simulink model "EMI_SC01B_R2_Halfbridge"  (R2026a)
settings: Solver=FixedStepDiscrete  StopTime=5.0000000000000004e-06  FixedStep=5.0000000000000003e-10  RelTol=1.0000000000000001e-05  AbsTol=1.0000000000000001e-09
model workspace (MAT data in the model file):
  sc01bGateHigh = timeseries
  sc01bGateHigh.Name = 'unnamed'
  sc01bGateHigh.DataInfo = tsdata.datametadata
  sc01bGateHigh.DataInfo.Interpolation = tsdata.interpolation
  sc01bGateHigh.DataInfo.Interpolation.Fhandle : function handle (value not decoded)
  sc01bGateHigh.DataInfo.Interpolation.Name = 'linear'
  sc01bGateHigh.TimeInfo = tsdata.timemetadata
  sc01bGateHigh.TimeInfo.Length = 10
  sc01bGateHigh.TimeInfo.DuplicateTimes = 0
  sc01bGateHigh.TimeInfo.Time_ = [0; 2.019e-06; 2.039e-06; 2.32e-06; 2.34e-06; 3.719e-06; 3.739e-06; 4.02e-06; 4.04e-06; 5e-06]
  sc01bGateHigh.TimeInfo.Initialized = 1
  sc01bGateHigh.QualityInfo = tsdata.qualmetadata
  sc01bGateHigh.Data_ = [12; 12; -1.5; -1.5; -1.5; -1.5; -1.5; -1.5; 12; 12]
  sc01bGateLow = timeseries
  sc01bGateLow.Name = 'unnamed'
  sc01bGateLow.DataInfo = tsdata.datametadata
  sc01bGateLow.DataInfo.Interpolation = tsdata.interpolation
  sc01bGateLow.DataInfo.Interpolation.Fhandle : function handle (value not decoded)
  sc01bGateLow.DataInfo.Interpolation.Name = 'linear'
  sc01bGateLow.TimeInfo = tsdata.timemetadata
  sc01bGateLow.TimeInfo.Length = 10
  sc01bGateLow.TimeInfo.DuplicateTimes = 0
  sc01bGateLow.TimeInfo.Time_ = [0; 2.019e-06; 2.039e-06; 2.32e-06; 2.34e-06; 3.719e-06; 3.739e-06; 4.02e-06; 4.04e-06; 5e-06]
  sc01bGateLow.TimeInfo.Initialized = 1
  sc01bGateLow.QualityInfo = tsdata.qualmetadata
  sc01bGateLow.Data_ = [-1.5; -1.5; -1.5; -1.5; 12; 12; -1.5; -1.5; -1.5; -1.5]
  sc01bParams.meta.id = "SC01B-R2-IAUC100N04S6L014"
  sc01bParams.meta.case = "nominal"
  sc01bParams.meta.scope = "Isothermal device-model verification; no physical source validation"
  sc01bParams.device.series = "Infineon OptiMOS6 40V"
  sc01bParams.device.name = "IAUC100N04S6L014"
  sc01bParams.device.temperature_C = 25
  sc01bParams.device.voltageRating_V = 40
  sc01bParams.device.gateRating_V = 16
  sc01bParams.device.source = "MATLAB R2026a shipped Infineon SPICE model, typical parameters"
  sc01bParams.bus.voltage_V = 24
  sc01bParams.bus.feedResistance_Ohm = 0.05
  sc01bParams.bus.feedInductance_H = 2e-08
  sc01bParams.bus.capacitance_F = 1e-05
  sc01bParams.bus.capacitorESR_Ohm = 0.01
  sc01bParams.bus.provenance = "Assumed bench supply and local decoupling, not selected layout or capacitor"
  sc01bParams.load.inductance_H = 0.0025
  sc01bParams.load.resistance_Ohm = 8
  sc01bParams.load.referenceCurrent_A = 3
  sc01bParams.load.provenance = "Assumed8ohm/2.5mH load; high-side initiallyON, consistentDC operating point near3A; current follows circuit equations"
  sc01bParams.driver.reference = "Revised bipolar behavioral driver with directional gate impedance; not UCC27211A-equivalent"
  sc01bParams.driver.voltage_V = 12
  sc01bParams.driver.outputResistance_Ohm = 3
  sc01bParams.driver.externalResistance_Ohm = 22
  sc01bParams.driver.additionalTurnOnResistance_Ohm = 0
  sc01bParams.driver.turnOffResistance_Ohm = 3
  sc01bParams.driver.offVoltage_V = -1.5
  sc01bParams.driver.riseDelay_s = 2e-08
  sc01bParams.driver.fallDelay_s = 1.9e-08
  sc01bParams.driver.commandRamp_s = 2e-08
  sc01bParams.driver.provenance = "R2 assumes 12V on/-1.5V off regulated floating supplies and unequal charge/discharge impedance. Ron=3ohm+external gate resistor; total Roff=3ohm. The original 20/19ns delays,20ns linear ramps,and300ns deadtime are retained. Negative rail and split-output behavior are explicit design changes; no complete driver IC, current limit, clamp diode dynamics, or bootstrap dynamics are modeled."
  sc01bParams.control.highOn_s = 4e-06
  sc01bParams.control.highOff_s = 2e-06
  sc01bParams.control.initialHigh = 1
  sc01bParams.control.deadTime_s = 3e-07
  sc01bParams.control.provenance = "Assumed high-side off/on commutation pair with complementary low-side operation; dead time commanded before driver delay"
  sc01bParams.simulation.stopTime_s = 5e-06
  sc01bParams.simulation.maxStep_s = 5e-10
  sc01bParams.simulation.relativeTolerance = 1e-05
  sc01bParams.simulation.absoluteTolerance = 1e-09
  sc01bParams.validation.startTime_s = 1e-06
  sc01bParams.validation.provenance = "Exclude initialization preamble from edge comparison; separately report initial and pre-edge current"
  sc01bSchema = 4
undefined symbols (not defined in the file): ee
libraries: fl_lib x24, nesl_utility x17, sc01b_driver_lib x2
settings Model: Creator=adand  LastModifiedBy=adand
settings DebuggingCC: MinStepSizeMsg=error
settings SimscapeCC: SimscapeLogName=sc01bSimlog  SimscapeLogLimitData=off

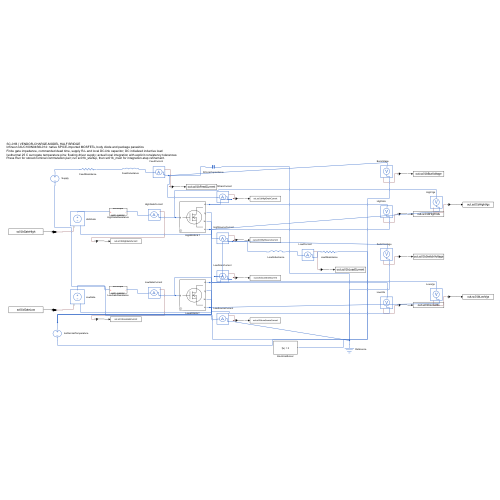
[thumbnail: Simulink's stored preview of the top-level diagram]
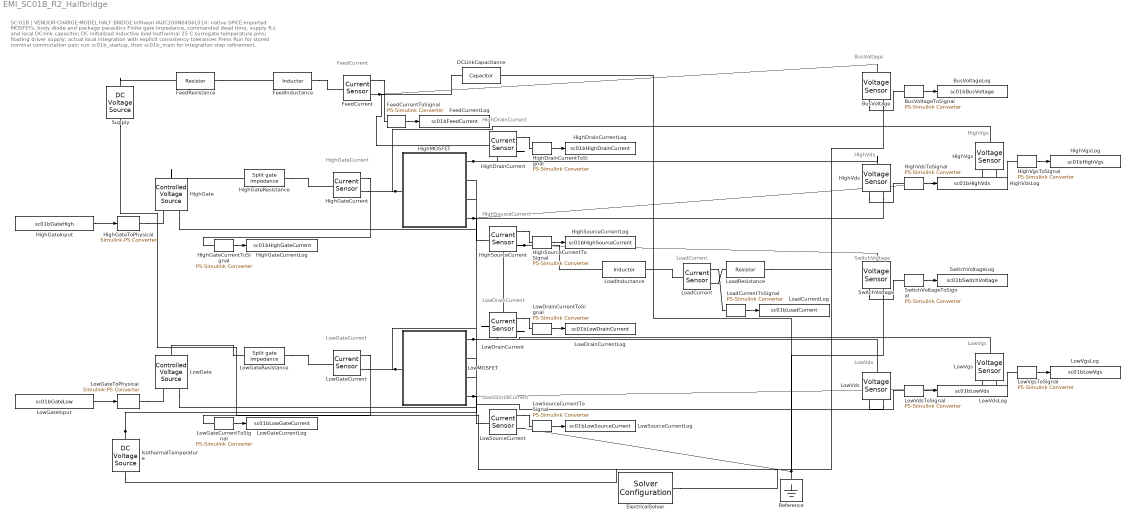
== system EMI_SC01B_R2_Halfbridge ==
  note: FeedCurrent
  note: HighDrainCurrent
  note: HighSourceCurrent
  note: LowDrainCurrent
  note: LowSourceCurrent
  note: HighGateCurrent
  note: LowGateCurrent
  note: LoadCurrent
  note: SwitchVoltage
  note: BusVoltage
  note: HighVgs
  note: HighVds
  note: LowVgs
  note: LowVds
  note: SC-01B | VENDOR-CHARGE-MODEL HALF BRIDGE
      | Infineon IAUC100N04S6L014: native SPICE-imported MOSFETs, body diode and package parasitics
      | Finite gate impedance, commanded dead time, supply R-L and local DC-link capacitor; DC initialized inductive load
      | Isothermal 25 C surrogate temperature pins; floating driver supply; actual local integration with explicit consistency tolerances
      | Press Run for stored nominal commutation pair; run sc01b_startup, then sc01b_main for integration-step refinement.
  BusVoltage : fl_lib/Electrical/Electrical Sensors/Voltage Sensor
  BusVoltageLog : ToWorkspace  VariableName=sc01bBusVoltage  SaveFormat=Timeseries  SampleTime=-1
  BusVoltageToSignal : nesl_utility/PS-Simulink Converter  PhysicalDomain=network_engine_domain  SubClassName=ps_output  LeftPortType=input  RightPortType=output  PseudoPeriodic=off  Frequencies=[]  VectorFormat=inherit  Unit=V  AffineConversion=off
  DCLinkCapacitance : fl_lib/Electrical/Electrical Elements/Capacitor  c=sc01bParams.bus.capacitance_F F  r=sc01bParams.bus.capacitorESR_Ohm Ohm  g=0 1/Ohm  i_specify=off  i_priority=None  i=0 A  i_nominal_specify=off  i_nominal_value=1  i_nominal_unit=A  v_specify=off  v_priority=None  v=0 V  v_nominal_specify=off  v_nominal_value=1  v_nominal_unit=V  vc_specify=off  vc_priority=High  vc=0 V  vc_nominal_specify=off  vc_nominal_value=1  vc_nominal_unit=V
  ElectricalSolver : nesl_utility/Solver Configuration  PhysicalDomain=network_engine_domain  SubClassName=solver  LeftPortType=input  RightPortType=generic  Tones=[]  Harmonics=[]  SimulateNoise=off  Profile=off  UseLocalSampling=off  EnableSwitchedLinearOptims=on  FrequencyDomain=off  UseCCode=off  RelTol=0.001  AbsTol=0.001  MinStep=1e-09  ToWorkspace=off  RevertToSquareIcSolve=off  NumHomotopyIterations=100  PhasorMode=off  PhasorModeNumHarmonics=1  ConsistencySolver=NEWTON_XTOL_AFTER_FTOL  CanonicalOrdering=CANONICAL  OptimizeIntermediates=OPTIMIZED  IndexReductionMethod=DerivativeReplacement  DoDC=on  ResidualTolerance=1e-09  ConsistencyTolSource=LOCAL  ConsistencyAbsTol=9.9999999999999998e-13  ConsistencyRelTol=1e-08  ConsistencyTolFactor=1  UseLocalSolver=on  LocalSolverChoice=NE_TRAPEZOIDAL_ADVANCER  ResolveIndetEquations=on  FunctionEvalNumThread=1  LocalSolverSampleTime=5.0000000000000003e-10  DoFixedCost=off  MaxNonlinIter=3  MaxModeIter=2  ComputeImpulses=off  ImpulseIterations=2  LinearAlgebra=auto  LinearAlgebraNumThread=0  EquationFormulation=NE_TIME_EF  DelaysMemoryBudget=1024  AutomaticFiltering=off  FilteringTimeConstant=0.001  PartitionStorageMethod=AS_NEEDED  PartitionMemoryBudget=1024  PartitionMethod=ROBUST  MultibodyUseLocalSolver=off  MultibodyLocalSolverChoice=ODE1  MultibodyLocalSolverSampleTime=0.001
  FeedCurrent : fl_lib/Electrical/Electrical Sensors/Current Sensor
  FeedCurrentLog : ToWorkspace  VariableName=sc01bFeedCurrent  SaveFormat=Timeseries  SampleTime=-1
  FeedCurrentToSignal : nesl_utility/PS-Simulink Converter  PhysicalDomain=network_engine_domain  SubClassName=ps_output  LeftPortType=input  RightPortType=output  PseudoPeriodic=off  Frequencies=[]  VectorFormat=inherit  Unit=A  AffineConversion=off
  FeedInductance : fl_lib/Electrical/Electrical Elements/Inductor  l=sc01bParams.bus.feedInductance_H H  r=0 Ohm  g=0 1/Ohm  i_specify=off  i_priority=None  i=0 A  i_nominal_specify=off  i_nominal_value=1  i_nominal_unit=A  v_specify=off  v_priority=None  v=0 V  v_nominal_specify=off  v_nominal_value=1  v_nominal_unit=V  i_L_specify=off  i_L_priority=High  i_L=0 A  i_L_nominal_specify=off  i_L_nominal_value=1  i_L_nominal_unit=A
  FeedResistance : fl_lib/Electrical/Electrical Elements/Resistor  R=sc01bParams.bus.feedResistance_Ohm Ohm  i_specify=off  i_priority=None  i=0 A  i_nominal_specify=off  i_nominal_value=1  i_nominal_unit=A  v_specify=off  v_priority=None  v=0 V  v_nominal_specify=off  v_nominal_value=1  v_nominal_unit=V
  HighDrainCurrent : fl_lib/Electrical/Electrical Sensors/Current Sensor
  HighDrainCurrentLog : ToWorkspace  VariableName=sc01bHighDrainCurrent  SaveFormat=Timeseries  SampleTime=-1
  HighDrainCurrentToSignal : nesl_utility/PS-Simulink Converter  PhysicalDomain=network_engine_domain  SubClassName=ps_output  LeftPortType=input  RightPortType=output  PseudoPeriodic=off  Frequencies=[]  VectorFormat=inherit  Unit=A  AffineConversion=off
  HighGate : fl_lib/Electrical/Electrical Sources/Controlled Voltage Source
  HighGateCurrent : fl_lib/Electrical/Electrical Sensors/Current Sensor
  HighGateCurrentLog : ToWorkspace  VariableName=sc01bHighGateCurrent  SaveFormat=Timeseries  SampleTime=-1
  HighGateCurrentToSignal : nesl_utility/PS-Simulink Converter  PhysicalDomain=network_engine_domain  SubClassName=ps_output  LeftPortType=input  RightPortType=output  PseudoPeriodic=off  Frequencies=[]  VectorFormat=inherit  Unit=A  AffineConversion=off
  HighGateInput : FromWorkspace  VariableName=sc01bGateHigh  OutputAfterFinalValue=Holding final value
  HighGateResistance : sc01b_driver_lib/Split gate impedance  Ron=sc01bParams.driver.outputResistance_Ohm+sc01bParams.driver.externalResistance_Ohm+sc01bParams.driver.additionalTurnOnResistance_Ohm Ohm  Roff=sc01bParams.driver.turnOffResistance_Ohm Ohm  i_specify=off  i_priority=None  i=0 A  i_nominal_specify=off  i_nominal_value=1  i_nominal_unit=A  v_specify=off  v_priority=None  v=0 V  v_nominal_specify=off  v_nominal_value=1  v_nominal_unit=V
  HighGateToPhysical : nesl_utility/Simulink-PS Converter  PhysicalDomain=network_engine_domain  SubClassName=ps_input  LeftPortType=input  RightPortType=output  PseudoPeriodic=off  Frequencies=[]  NoiseDistribution=none  NoiseParameters=[]  Unit=V  AffineConversion=off  FilteringAndDerivatives=provide  SimscapeFilterOrder=1  InputFilterTimeConstant=0.001  UdotUserProvided=0
  HighMOSFET : Subsystem  LoadFcn=ee.forwardingCallback();  mask(SPICE-Imported MOSFET){SeriesChoice=Infineon OptiMOS6 40V, DeviceChoice=IAUC100N04S6L014}
      mask prompts: SeriesChoice "physmod:ee:spiceimportedmosfet:Series_MP"; DeviceChoice "physmod:ee:spiceimportedmosfet:Device_MP"
      mask help: physmod:ee:spiceimportedmosfet:SPICEimportedMOSFETblock_MD
      mask init:
      | ee.internal.spice.maskInitialization(gcb)
      settings: CopyFcn=set_param(gcb,'LinkStatus','none');
      mask Help: helpview('sps','spice-imported-mosfet-block')
      mask TypeOptions SeriesChoice: Infineon OptiMOS7 40V | Infineon OptiMOS6 40V | Infineon OptiMOS5 60V | Infineon OptiMOS4 60V | Infineon OptiMOS7 80V | Infineon OptiMOS5 80V | Infineon OptiMOS7 100V | Infineon OptiMOS5 100V | Infineon OptiMOS5 120V | Infineon OptiMOST 120V
      mask Callback SeriesChoice:
      | %Run mask initialization to update the block help
      | ee.internal.spice.seriesCallback(gcb)
      mask TypeOptions DeviceChoice: IAUC60N04S6L039 | IAUC60N04S6N044 | IAUC80N04S6L032 | IAUC80N04S6N036 | IAUC100N04S6L014 | IAUC100N04S6L020 | IAUC100N04S6L025 | IAUC100N04S6N015 | IAUC100N04S6N022 | IAUC100N04S6N028 | IAUC120N04S6L008 | IAUC120N04S6L009 | IAUC120N04S6L012 | IAUC120N04S6N009 | IAUC120N04S6N010 | IAUC120N04S6N013
      mask DialogControl ParameterGroupVar Prompt: physmod:ee:spiceimportedmosfet:DeviceSelection_MH
      mask DialogControl SeriesChoice Prompt: Series
      mask DialogControl DeviceChoice Prompt: Device
  HighSourceCurrent : fl_lib/Electrical/Electrical Sensors/Current Sensor
  HighSourceCurrentLog : ToWorkspace  VariableName=sc01bHighSourceCurrent  SaveFormat=Timeseries  SampleTime=-1
  HighSourceCurrentToSignal : nesl_utility/PS-Simulink Converter  PhysicalDomain=network_engine_domain  SubClassName=ps_output  LeftPortType=input  RightPortType=output  PseudoPeriodic=off  Frequencies=[]  VectorFormat=inherit  Unit=A  AffineConversion=off
  HighVds : fl_lib/Electrical/Electrical Sensors/Voltage Sensor
  HighVdsLog : ToWorkspace  VariableName=sc01bHighVds  SaveFormat=Timeseries  SampleTime=-1
  HighVdsToSignal : nesl_utility/PS-Simulink Converter  PhysicalDomain=network_engine_domain  SubClassName=ps_output  LeftPortType=input  RightPortType=output  PseudoPeriodic=off  Frequencies=[]  VectorFormat=inherit  Unit=V  AffineConversion=off
  HighVgs : fl_lib/Electrical/Electrical Sensors/Voltage Sensor
  HighVgsLog : ToWorkspace  VariableName=sc01bHighVgs  SaveFormat=Timeseries  SampleTime=-1
  HighVgsToSignal : nesl_utility/PS-Simulink Converter  PhysicalDomain=network_engine_domain  SubClassName=ps_output  LeftPortType=input  RightPortType=output  PseudoPeriodic=off  Frequencies=[]  VectorFormat=inherit  Unit=V  AffineConversion=off
  IsothermalTemperature : fl_lib/Electrical/Electrical Sources/DC Voltage Source  v0=sc01bParams.device.temperature_C V
  LoadCurrent : fl_lib/Electrical/Electrical Sensors/Current Sensor
  LoadCurrentLog : ToWorkspace  VariableName=sc01bLoadCurrent  SaveFormat=Timeseries  SampleTime=-1
  LoadCurrentToSignal : nesl_utility/PS-Simulink Converter  PhysicalDomain=network_engine_domain  SubClassName=ps_output  LeftPortType=input  RightPortType=output  PseudoPeriodic=off  Frequencies=[]  VectorFormat=inherit  Unit=A  AffineConversion=off
  LoadInductance : fl_lib/Electrical/Electrical Elements/Inductor  l=sc01bParams.load.inductance_H H  r=0 Ohm  g=0 1/Ohm  i_specify=off  i_priority=None  i=0 A  i_nominal_specify=off  i_nominal_value=1  i_nominal_unit=A  v_specify=off  v_priority=None  v=0 V  v_nominal_specify=off  v_nominal_value=1  v_nominal_unit=V  i_L_specify=off  i_L_priority=High  i_L=0 A  i_L_nominal_specify=off  i_L_nominal_value=1  i_L_nominal_unit=A
  LoadResistance : fl_lib/Electrical/Electrical Elements/Resistor  R=sc01bParams.load.resistance_Ohm Ohm  i_specify=off  i_priority=None  i=0 A  i_nominal_specify=off  i_nominal_value=1  i_nominal_unit=A  v_specify=off  v_priority=None  v=0 V  v_nominal_specify=off  v_nominal_value=1  v_nominal_unit=V
  LowDrainCurrent : fl_lib/Electrical/Electrical Sensors/Current Sensor
  LowDrainCurrentLog : ToWorkspace  VariableName=sc01bLowDrainCurrent  SaveFormat=Timeseries  SampleTime=-1
  LowDrainCurrentToSignal : nesl_utility/PS-Simulink Converter  PhysicalDomain=network_engine_domain  SubClassName=ps_output  LeftPortType=input  RightPortType=output  PseudoPeriodic=off  Frequencies=[]  VectorFormat=inherit  Unit=A  AffineConversion=off
  LowGate : fl_lib/Electrical/Electrical Sources/Controlled Voltage Source
  LowGateCurrent : fl_lib/Electrical/Electrical Sensors/Current Sensor
  LowGateCurrentLog : ToWorkspace  VariableName=sc01bLowGateCurrent  SaveFormat=Timeseries  SampleTime=-1
  LowGateCurrentToSignal : nesl_utility/PS-Simulink Converter  PhysicalDomain=network_engine_domain  SubClassName=ps_output  LeftPortType=input  RightPortType=output  PseudoPeriodic=off  Frequencies=[]  VectorFormat=inherit  Unit=A  AffineConversion=off
  LowGateInput : FromWorkspace  VariableName=sc01bGateLow  OutputAfterFinalValue=Holding final value
  LowGateResistance : sc01b_driver_lib/Split gate impedance  Ron=sc01bParams.driver.outputResistance_Ohm+sc01bParams.driver.externalResistance_Ohm+sc01bParams.driver.additionalTurnOnResistance_Ohm Ohm  Roff=sc01bParams.driver.turnOffResistance_Ohm Ohm  i_specify=off  i_priority=None  i=0 A  i_nominal_specify=off  i_nominal_value=1  i_nominal_unit=A  v_specify=off  v_priority=None  v=0 V  v_nominal_specify=off  v_nominal_value=1  v_nominal_unit=V
  LowGateToPhysical : nesl_utility/Simulink-PS Converter  PhysicalDomain=network_engine_domain  SubClassName=ps_input  LeftPortType=input  RightPortType=output  PseudoPeriodic=off  Frequencies=[]  NoiseDistribution=none  NoiseParameters=[]  Unit=V  AffineConversion=off  FilteringAndDerivatives=provide  SimscapeFilterOrder=1  InputFilterTimeConstant=0.001  UdotUserProvided=0
  LowMOSFET : Subsystem  LoadFcn=ee.forwardingCallback();  mask(SPICE-Imported MOSFET){SeriesChoice=Infineon OptiMOS6 40V, DeviceChoice=IAUC100N04S6L014}
      mask prompts: SeriesChoice "physmod:ee:spiceimportedmosfet:Series_MP"; DeviceChoice "physmod:ee:spiceimportedmosfet:Device_MP"
      mask help: physmod:ee:spiceimportedmosfet:SPICEimportedMOSFETblock_MD
      mask init:
      | ee.internal.spice.maskInitialization(gcb)
      settings: CopyFcn=set_param(gcb,'LinkStatus','none');
      mask Help: helpview('sps','spice-imported-mosfet-block')
      mask TypeOptions SeriesChoice: Infineon OptiMOS7 40V | Infineon OptiMOS6 40V | Infineon OptiMOS5 60V | Infineon OptiMOS4 60V | Infineon OptiMOS7 80V | Infineon OptiMOS5 80V | Infineon OptiMOS7 100V | Infineon OptiMOS5 100V | Infineon OptiMOS5 120V | Infineon OptiMOST 120V
      mask Callback SeriesChoice:
      | %Run mask initialization to update the block help
      | ee.internal.spice.seriesCallback(gcb)
      mask TypeOptions DeviceChoice: IAUC60N04S6L039 | IAUC60N04S6N044 | IAUC80N04S6L032 | IAUC80N04S6N036 | IAUC100N04S6L014 | IAUC100N04S6L020 | IAUC100N04S6L025 | IAUC100N04S6N015 | IAUC100N04S6N022 | IAUC100N04S6N028 | IAUC120N04S6L008 | IAUC120N04S6L009 | IAUC120N04S6L012 | IAUC120N04S6N009 | IAUC120N04S6N010 | IAUC120N04S6N013
      mask DialogControl ParameterGroupVar Prompt: physmod:ee:spiceimportedmosfet:DeviceSelection_MH
      mask DialogControl SeriesChoice Prompt: Series
      mask DialogControl DeviceChoice Prompt: Device
  LowSourceCurrent : fl_lib/Electrical/Electrical Sensors/Current Sensor
  LowSourceCurrentLog : ToWorkspace  VariableName=sc01bLowSourceCurrent  SaveFormat=Timeseries  SampleTime=-1
  LowSourceCurrentToSignal : nesl_utility/PS-Simulink Converter  PhysicalDomain=network_engine_domain  SubClassName=ps_output  LeftPortType=input  RightPortType=output  PseudoPeriodic=off  Frequencies=[]  VectorFormat=inherit  Unit=A  AffineConversion=off
  LowVds : fl_lib/Electrical/Electrical Sensors/Voltage Sensor
  LowVdsLog : ToWorkspace  VariableName=sc01bLowVds  SaveFormat=Timeseries  SampleTime=-1
  LowVdsToSignal : nesl_utility/PS-Simulink Converter  PhysicalDomain=network_engine_domain  SubClassName=ps_output  LeftPortType=input  RightPortType=output  PseudoPeriodic=off  Frequencies=[]  VectorFormat=inherit  Unit=V  AffineConversion=off
  LowVgs : fl_lib/Electrical/Electrical Sensors/Voltage Sensor
  LowVgsLog : ToWorkspace  VariableName=sc01bLowVgs  SaveFormat=Timeseries  SampleTime=-1
  LowVgsToSignal : nesl_utility/PS-Simulink Converter  PhysicalDomain=network_engine_domain  SubClassName=ps_output  LeftPortType=input  RightPortType=output  PseudoPeriodic=off  Frequencies=[]  VectorFormat=inherit  Unit=V  AffineConversion=off
  Reference : fl_lib/Electrical/Electrical Elements/Electrical Reference
  Supply : fl_lib/Electrical/Electrical Sources/DC Voltage Source  v0=sc01bParams.bus.voltage_V V
  SwitchVoltage : fl_lib/Electrical/Electrical Sensors/Voltage Sensor
  SwitchVoltageLog : ToWorkspace  VariableName=sc01bSwitchVoltage  SaveFormat=Timeseries  SampleTime=-1
  SwitchVoltageToSignal : nesl_utility/PS-Simulink Converter  PhysicalDomain=network_engine_domain  SubClassName=ps_output  LeftPortType=input  RightPortType=output  PseudoPeriodic=off  Frequencies=[]  VectorFormat=inherit  Unit=V  AffineConversion=off
  wires:
  HighGateInput/1 -> HighGateToPhysical/1
  LowGateInput/1 -> LowGateToPhysical/1
  FeedCurrentToSignal/1 -> FeedCurrentLog/1
  HighDrainCurrentToSignal/1 -> HighDrainCurrentLog/1
  HighSourceCurrentToSignal/1 -> HighSourceCurrentLog/1
  LowDrainCurrentToSignal/1 -> LowDrainCurrentLog/1
  LowSourceCurrentToSignal/1 -> LowSourceCurrentLog/1
  HighGateCurrentToSignal/1 -> HighGateCurrentLog/1
  LowGateCurrentToSignal/1 -> LowGateCurrentLog/1
  LoadCurrentToSignal/1 -> LoadCurrentLog/1
  SwitchVoltageToSignal/1 -> SwitchVoltageLog/1
  BusVoltageToSignal/1 -> BusVoltageLog/1
  HighVgsToSignal/1 -> HighVgsLog/1
  HighVdsToSignal/1 -> HighVdsLog/1
  LowVgsToSignal/1 -> LowVgsLog/1
  LowVdsToSignal/1 -> LowVdsLog/1
  connections:
  HighGateToPhysical/RConn1 -- HighGate/RConn1
  LowGateToPhysical/RConn1 -- LowGate/RConn1
  FeedCurrent/RConn1 -- FeedCurrentToSignal/LConn1
  HighDrainCurrent/RConn1 -- HighDrainCurrentToSignal/LConn1
  HighSourceCurrent/RConn1 -- HighSourceCurrentToSignal/LConn1
  LowDrainCurrent/RConn1 -- LowDrainCurrentToSignal/LConn1
  LowSourceCurrent/RConn1 -- LowSourceCurrentToSignal/LConn1
  HighGateCurrent/RConn1 -- HighGateCurrentToSignal/LConn1
  LowGateCurrent/RConn1 -- LowGateCurrentToSignal/LConn1
  LoadCurrent/RConn1 -- LoadCurrentToSignal/LConn1
  SwitchVoltage/RConn1 -- SwitchVoltageToSignal/LConn1
  BusVoltage/RConn1 -- BusVoltageToSignal/LConn1
  HighVgs/RConn1 -- HighVgsToSignal/LConn1
  HighVds/RConn1 -- HighVdsToSignal/LConn1
  LowVgs/RConn1 -- LowVgsToSignal/LConn1
  LowVds/RConn1 -- LowVdsToSignal/LConn1
  Supply/LConn1 -- FeedResistance/LConn1
  FeedResistance/RConn1 -- FeedInductance/LConn1
  FeedInductance/RConn1 -- FeedCurrent/LConn1
  DCLinkCapacitance/LConn1 -- FeedCurrent/RConn2 -- HighDrainCurrent/LConn1 -- BusVoltage/LConn1
  DCLinkCapacitance/RConn1 -- Reference/LConn1 -- LowSourceCurrent/RConn2 -- LoadResistance/RConn1 -- Supply/RConn1 -- IsothermalTemperature/RConn1 -- ElectricalSolver/RConn1 -- SwitchVoltage/RConn2 -- BusVoltage/RConn2
  HighMOSFET/RConn1 -- HighDrainCurrent/RConn2 -- HighVds/LConn1
  HighSourceCurrent/LConn1 -- HighMOSFET/RConn4 -- HighGate/RConn2 -- HighVgs/RConn2 -- HighVds/RConn2
  LowDrainCurrent/LConn1 -- HighSourceCurrent/RConn2 -- LoadInductance/LConn1 -- SwitchVoltage/LConn1
  LowMOSFET/RConn1 -- LowDrainCurrent/RConn2 -- LowVds/LConn1
  LowSourceCurrent/LConn1 -- LowMOSFET/RConn4 -- LowGate/RConn2 -- LowVgs/RConn2 -- LowVds/RConn2
  LoadInductance/RConn1 -- LoadCurrent/LConn1
  LoadCurrent/RConn2 -- LoadResistance/LConn1
  HighGate/LConn1 -- HighGateResistance/LConn1
  HighGateResistance/RConn1 -- HighGateCurrent/LConn1
  HighMOSFET/LConn1 -- HighGateCurrent/RConn2 -- HighVgs/LConn1
  HighMOSFET/RConn2 -- IsothermalTemperature/LConn1 -- HighMOSFET/RConn3 -- LowMOSFET/RConn2 -- LowMOSFET/RConn3
  LowGate/LConn1 -- LowGateResistance/LConn1
  LowGateResistance/RConn1 -- LowGateCurrent/LConn1
  LowMOSFET/LConn1 -- LowGateCurrent/RConn2 -- LowVgs/LConn1

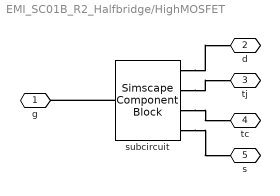
== system EMI_SC01B_R2_Halfbridge/HighMOSFET ==
  subcircuit : SimscapeComponentBlock  SourceFile=ee_spice_mosfets.spiceinfineon.spiceOptiMOS_6_40V.IAUC100N04S6L014  ComponentPath=ee_spice_mosfets.spiceinfineon.spiceOptiMOS_6_40V.IAUC100N04S6L014  ComponentVariants="[\"ee_spice_mosfets.spiceinfineon.spiceOptiMOS_6_40V.IAUC100N04S6L014\"]"  ComponentVariantNames="[\"IAUC100N04S6L014\"]"  ClassName=IAUC100N04S6L014  SchemaVersion=1  dvth=0  drdson=0  dgfs=0  dc=0  dzth=0  ls=5e-11  ld=1e-09  lg=3e-09  specifyParasiticValues=ee.enum.include.yes  capacitorSeriesResistance=1e-07 Ohm  inductorParallelConductance=1e-07 1/Ohm  specifySmoothValues=ee.enum.include.no  aWarning=ee.enum.include.no  crossZero=ee.enum.include.no  dropPowerFlag=ee.enum.function.powerFlag.hyp  dropPowerHypEpsilon=0  expXh=Inf  expXl=-Inf  logX0=0  smoothEpsilon=0  smoothN=1  G_S_specify=off  G_S_priority=None  G_S=0 A  G_S_nominal_specify=off  G_S_nominal_value=1  G_S_nominal_unit=A
      settings: CopyFcn=simscape.sscblock.internal.componentBlockCallback(gcbh,'COPY')  PreCopyFcn=simscape.sscblock.internal.componentBlockCallback(gcbh,'PRECOPY')  PreDeleteFcn=simscape.sscblock.internal.componentBlockCallback(gcbh,'PREDELETE')
      mask Type: IAUC100N04S6L014
  g : PMIOPort  Side=Left
  d : PMIOPort  Port=2  Side=Right
  tj : PMIOPort  Port=3  Side=Right
  tc : PMIOPort  Port=4  Side=Right
  s : PMIOPort  Port=5  Side=Right
  connections:
  subcircuit/RConn4 -- s/RConn1
  subcircuit/RConn3 -- tc/RConn1
  subcircuit/RConn2 -- tj/RConn1
  subcircuit/RConn1 -- d/RConn1
  subcircuit/LConn1 -- g/RConn1

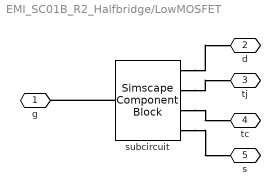
== system EMI_SC01B_R2_Halfbridge/LowMOSFET ==
  subcircuit : SimscapeComponentBlock  SourceFile=ee_spice_mosfets.spiceinfineon.spiceOptiMOS_6_40V.IAUC100N04S6L014  ComponentPath=ee_spice_mosfets.spiceinfineon.spiceOptiMOS_6_40V.IAUC100N04S6L014  ComponentVariants="[\"ee_spice_mosfets.spiceinfineon.spiceOptiMOS_6_40V.IAUC100N04S6L014\"]"  ComponentVariantNames="[\"IAUC100N04S6L014\"]"  ClassName=IAUC100N04S6L014  SchemaVersion=1  dvth=0  drdson=0  dgfs=0  dc=0  dzth=0  ls=5e-11  ld=1e-09  lg=3e-09  specifyParasiticValues=ee.enum.include.yes  capacitorSeriesResistance=1e-07 Ohm  inductorParallelConductance=1e-07 1/Ohm  specifySmoothValues=ee.enum.include.no  aWarning=ee.enum.include.no  crossZero=ee.enum.include.no  dropPowerFlag=ee.enum.function.powerFlag.hyp  dropPowerHypEpsilon=0  expXh=Inf  expXl=-Inf  logX0=0  smoothEpsilon=0  smoothN=1  G_S_specify=off  G_S_priority=None  G_S=0 A  G_S_nominal_specify=off  G_S_nominal_value=1  G_S_nominal_unit=A
      settings: CopyFcn=simscape.sscblock.internal.componentBlockCallback(gcbh,'COPY')  PreCopyFcn=simscape.sscblock.internal.componentBlockCallback(gcbh,'PRECOPY')  PreDeleteFcn=simscape.sscblock.internal.componentBlockCallback(gcbh,'PREDELETE')
      mask Type: IAUC100N04S6L014
  g : PMIOPort  Side=Left
  d : PMIOPort  Port=2  Side=Right
  tj : PMIOPort  Port=3  Side=Right
  tc : PMIOPort  Port=4  Side=Right
  s : PMIOPort  Port=5  Side=Right
  connections:
  subcircuit/RConn4 -- s/RConn1
  subcircuit/RConn3 -- tc/RConn1
  subcircuit/RConn2 -- tj/RConn1
  subcircuit/RConn1 -- d/RConn1
  subcircuit/LConn1 -- g/RConn1
